simulink model "tutorial07_subsystem"  (R2025a)
settings: Solver=VariableStepAuto  StartTime=0.0  StopTime=10.0  RelTol=1e-3
settings Model: Creator=xing2  LastModifiedBy=xing2

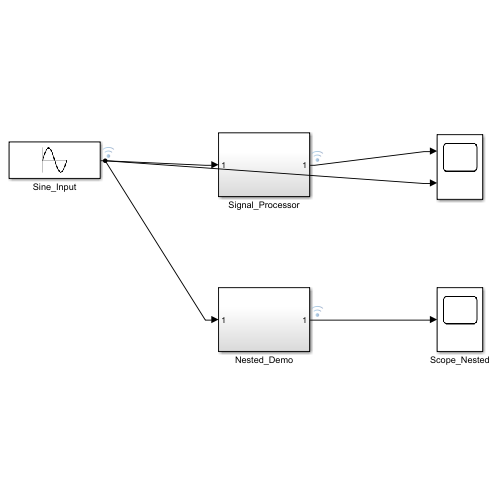
[thumbnail: Simulink's stored preview of the top-level diagram]
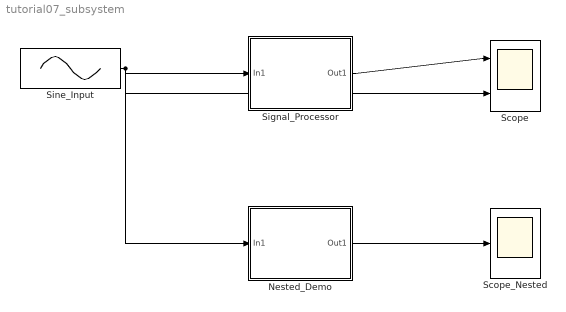
== system tutorial07_subsystem ==
  Nested_Demo : Subsystem
  Scope : Scope  NumInputPorts=2
  Scope_Nested : Scope
  Signal_Processor : Subsystem
  Sine_Input : Sin  Amplitude=5  SampleTime=0
  wires:
  Sine_Input/1 -> Signal_Processor/1(In1), Scope/2, Nested_Demo/1(In1)
  Signal_Processor/1(Out1) -> Scope/1
  Nested_Demo/1(Out1) -> Scope_Nested/1

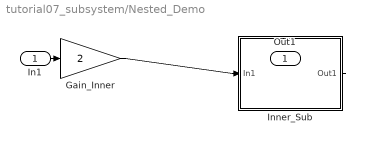
== system tutorial07_subsystem/Nested_Demo ==
  In1 : Inport
  Gain_Inner : Gain  Gain=2
  Inner_Sub : Subsystem
  Out1 : Outport
  wires:
  In1/1 -> Gain_Inner/1
  Gain_Inner/1 -> Inner_Sub/1(In1)
  Inner_Sub/1(Out1) -> Out1/1

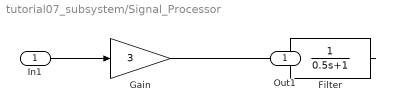
== system tutorial07_subsystem/Signal_Processor ==
  In1 : Inport
  Filter : TransferFcn  Denominator=[0.5 1]
  Gain : Gain  Gain=3
  Out1 : Outport
  wires:
  In1/1 -> Gain/1
  Gain/1 -> Filter/1
  Filter/1 -> Out1/1

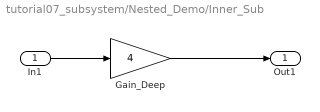
== system tutorial07_subsystem/Nested_Demo/Inner_Sub ==
  In1 : Inport
  Gain_Deep : Gain  Gain=4
      settings: AttributesFormatString=第3层！\nGain=4
  Out1 : Outport
  wires:
  In1/1 -> Gain_Deep/1
  Gain_Deep/1 -> Out1/1
